simulink model "fm"  (R2023b)
settings: Solver=FixedStepAuto  StartTime=0.0  StopTime=1  FixedStep=1e-5  RelTol=1e-3
libraries: dspfdesign x1, simulink x1
settings Model: Creator=B03-304  LastModifiedBy=B03-304

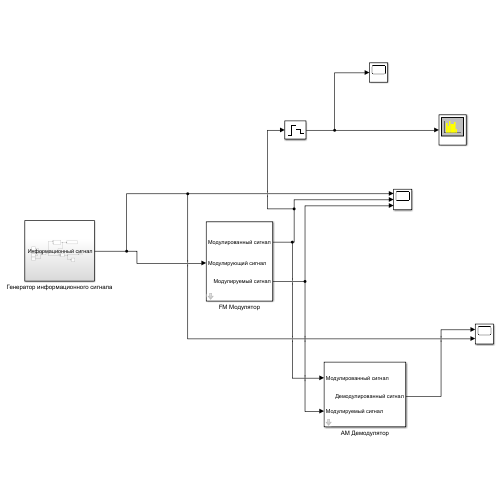
[thumbnail: Simulink's stored preview of the top-level diagram]
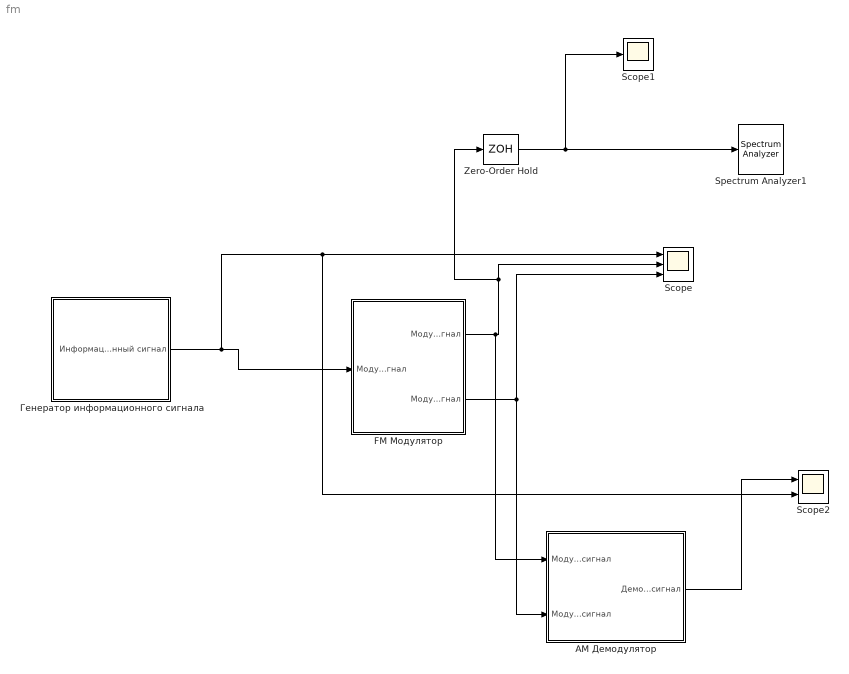
== system fm ==
  AM Демодулятор : Subsystem  mask{f0=300, m=0.7}
      mask prompts: f0 "Частота несущей"; m "Порядок модуляции"
  FM Модулятор : Subsystem  mask{f0=300, fd=100}
      mask prompts: f0 "Частота несущей"; fd "Девиация частоты"
  Scope : Scope  NumInputPorts=3
  Scope1 : Scope
  Scope2 : Scope  NumInputPorts=2
  Spectrum Analyzer1 : SpectrumAnalyzer  WindowPosition=[968.000000,406.000000,800.000000,500.000000,]  Visible=on  ScopeFrameLocation=window  PlotAsTwoSidedSpectrum=off  Span=5000  CenterFrequency=2500  StartFrequency=0  YLimits=[-160.10399317,-12.96289243]  SelectedToolstripTab=spectrumAnalyzerToolstrip.spectrumTab
  Zero-Order Hold : ZeroOrderHold  SampleTime=0.0001
  Генератор информационного сигнала : Subsystem
  wires:
  Zero-Order Hold/1 -> Spectrum Analyzer1/1, Scope1/1
  AM Демодулятор/1(Демодулированный сигнал) -> Scope2/1
  Генератор информационного сигнала/1(Информационный сигнал) -> Scope2/2, Scope/1, FM Модулятор/1(Модулирующий сигнал)
  FM Модулятор/1(Модулированный сигнал) -> AM Демодулятор/1(Модулированный сигнал), Zero-Order Hold/1, Scope/2
  FM Модулятор/2(Модулируемый сигнал) -> AM Демодулятор/2(Модулируемый сигнал), Scope/3

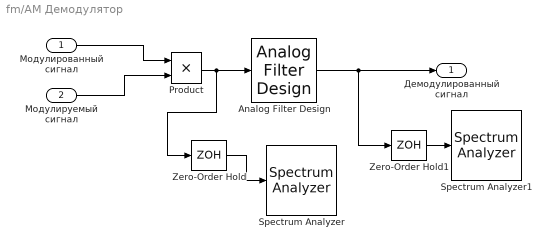
== system fm/AM Демодулятор ==
  Модулированный сигнал : Inport
  Модулируемый сигнал : Inport  Port=2
  Analog Filter Design : dspfdesign/Analog Filter Design  method=Butterworth  filttype=Lowpass  N=16  Wlo=f0*2*pi  Whi=80  Rp=2  Rs=40
  Product : Product
  Spectrum Analyzer : SpectrumAnalyzer  Tag=simrfV2util1/Spectrum Analyzer  WindowPosition=[310.000000,573.000000,800.000000,500.000000,]  Visible=on  ScopeFrameLocation=window  Method=Welch  PlotAsTwoSidedSpectrum=off  Span=49999.99999999999  CenterFrequency=24999.999999999996  StartFrequency=0  StopFrequency=49999.99999999999  AveragingMethod=Exponential  YLimits=[-232.7665104,49.02334608]  SelectedToolstripTab=spectrumAnalyzerToolstrip.spectrumTab
  Spectrum Analyzer1 : SpectrumAnalyzer  Tag=simrfV2util1/Spectrum Analyzer  WindowPosition=[447.000000,256.000000,800.000000,500.000000,]  Visible=on  ScopeFrameLocation=window  Method=Welch  PlotAsTwoSidedSpectrum=off  Span=49999.99999999999  CenterFrequency=24999.999999999996  StartFrequency=0  StopFrequency=49999.99999999999  AveragingMethod=Exponential  YLimits=[-259.53465023,51.9486356]  SelectedToolstripTab=spectrumAnalyzerToolstrip.spectrumTab
  Zero-Order Hold : ZeroOrderHold  SampleTime=-1
  Zero-Order Hold1 : ZeroOrderHold  SampleTime=-1
  Демодулированный сигнал : Outport
  wires:
  Модулированный сигнал/1 -> Product/1
  Модулируемый сигнал/1 -> Product/2
  Product/1 -> Zero-Order Hold/1, Analog Filter Design/1
  Analog Filter Design/1 -> Zero-Order Hold1/1, Демодулированный сигнал/1
  Zero-Order Hold/1 -> Spectrum Analyzer/1
  Zero-Order Hold1/1 -> Spectrum Analyzer1/1

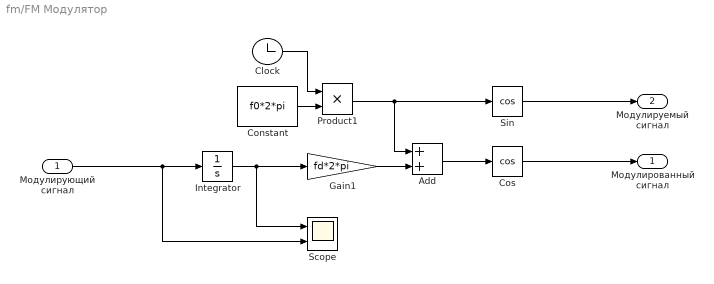
== system fm/FM Модулятор ==
  Модулирующий сигнал : Inport
  Add : Sum
  Clock : Clock
  Constant : Constant  Value=f0*2*pi
  Cos : Trigonometry  Operator=cos
  Gain1 : Gain  Gain=fd*2*pi
  Integrator : Integrator
  Product1 : Product
  Scope : Scope  NumInputPorts=2
  Sin : Trigonometry  Operator=cos
  Модулированный сигнал : Outport
  Модулируемый сигнал : Outport  Port=2
  wires:
  Cos/1 -> Модулированный сигнал/1
  Gain1/1 -> Add/2
  Add/1 -> Cos/1
  Constant/1 -> Product1/2
  Clock/1 -> Product1/1
  Product1/1 -> Add/1, Sin/1
  Модулирующий сигнал/1 -> Scope/2, Integrator/1
  Integrator/1 -> Gain1/1, Scope/1
  Sin/1 -> Модулируемый сигнал/1

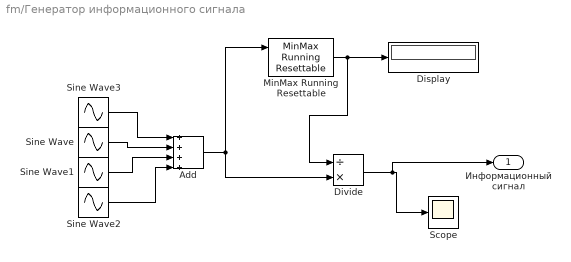
== system fm/Генератор информационного сигнала ==
  Add : Sum  Inputs=++++
  Display : Display
  Divide : Product  Inputs=/*
  MinMax Running Resettable : simulink/Math Operations/MinMax Running Resettable  Function=max  vinit=0.1
  Scope : Scope
  Sine Wave : Sin  Frequency=80*2*pi  SampleTime=0
  Sine Wave1 : Sin  Frequency=60*2*pi  SampleTime=0
  Sine Wave2 : Sin  Frequency=40*2*pi  SampleTime=0
  Sine Wave3 : Sin  Frequency=100*2*pi  SampleTime=0
  Информационный сигнал : Outport
  wires:
  Sine Wave3/1 -> Add/1
  Sine Wave/1 -> Add/2
  Sine Wave1/1 -> Add/3
  Sine Wave2/1 -> Add/4
  Add/1 -> MinMax Running Resettable/1, Divide/2
  MinMax Running Resettable/1 -> Divide/1, Display/1
  Divide/1 -> Информационный сигнал/1, Scope/1
